simulink model "BaseEngineController_LS"  (Simulink 7.7)
settings: Solver=FixedStepDiscrete  StartTime=0.0  StopTime=10.0  RelTol=1e-3
PreLoadFcn:
  | try, eval([bdroot '_setup']); catch, eval('model_setup', ''); end
InitFcn:
  | try, eval([bdroot '_setup']); catch, eval('model_setup', ''); end
undefined symbols (not defined in the file): ECU555, High, motohawk_build_version, motohawk_trunc_name, motohawk_vardec_config_group, motohawk_vardec_path, True
libraries: MotoHawk_lib x1418, motohawk_control_primitives_lib x183, motohawk_engine_lib x32, simulink x21, motohawk_annotations_lib x9, AutoDoc_lib x8, simulink_extras x4, motohawk_ccp_examples_lib x1, motohawk_control_primitives_motoshare_lib x1
(part 6 of 27)

== system BaseEngineController_LS/Foreground/Control/Diagnostics/MAP Fault Logic ==
  Sensors : Inport
  Add : Sum  Inputs=+-
  Bus Selector : BusSelector  OutputSignals=RawProcessed.EngineState
  Bus Selector1 : BusSelector  OutputSignals=RawProcessed.TPS
  Bus Selector2 : BusSelector  OutputSignals=RawProcessed.TPS
  Bus Selector3 : BusSelector  OutputSignals=RawProcessed.TPS
  Bus Selector4 : BusSelector  OutputSignals=Raw.LinearSensors.MAP_Angular
  Bus Selector5 : BusSelector  OutputSignals=Raw.LinearSensors.MAP_Angular
  Bus Selector6 : BusSelector  OutputSignals=AirCalcs.Baro,Raw.LinearSensors.MAP_Angular
  Logical Operator1 : Logic  Operator=OR  Inputs=6  AllPortsSameDT=off  OutDataTypeStr=boolean
  Logical Operator2 : Logic  Inputs=4  AllPortsSameDT=off  OutDataTypeStr=boolean
  Logical Operator3 : Logic  Operator=NOT  Inputs=3  AllPortsSameDT=off  OutDataTypeStr=boolean
  Logical Operator4 : Logic  Inputs=4  AllPortsSameDT=off  OutDataTypeStr=boolean
  Logical Operator5 : Logic  Inputs=4  AllPortsSameDT=off  OutDataTypeStr=boolean
  Relational Operator1 : RelationalOperator  Operator=>  OutDataTypeStr=boolean
  Relational Operator{2..3,7..8} (4 alike) : RelationalOperator  Operator=<  OutDataTypeStr=boolean
  Relational Operator4 : RelationalOperator  Operator=>  OutDataTypeStr=boolean
  Run State : motohawk_control_primitives_lib/CompareTo  SystemSampleTime=-1  op===  val=3
  motohawk_calibration2 : MotoHawk_lib/Calibration & Probing Blocks/motohawk_calibration  nam='MAP_IR_TPS_CL'  val=50  storage=Calibration  show_more=on  name_source=Use Parameter  data_type=double  read_level=1  write_level=1  ovr_cals=on  view_as=Number  enum_struct={'Disabled', 'Enabled'}  vector_style=Wide Row  use_help_units=on  help="'In-range MAP fault logic.  Maximum throttle position, below which MAP should be less than MAP_IR_HI'"  units='%'  use_header_enum=off  row_header_enum={}  col_header_enum={}  use_min_max=off  min_val=0  max_val=inf  use_precision=off  precision=''  gain=1  offset=0  exp=1  use_mototune_group=on  mototune_group=motohawk_vardec_path(gcb)
  motohawk_calibration4 : MotoHawk_lib/Calibration & Probing Blocks/motohawk_calibration  nam='MAP_IR_HI'  val=50  storage=Calibration  show_more=on  name_source=Use Parameter  data_type=double  read_level=1  write_level=1  ovr_cals=on  view_as=Number  enum_struct={'Disabled', 'Enabled'}  vector_style=Wide Row  use_help_units=on  help='In-range MAP fault logic. Maximum value that MAP should not exceed with closed throttle and engine running'  units='kPa'  use_header_enum=off  row_header_enum={}  col_header_enum={}  use_min_max=off  min_val=0  max_val=inf  use_precision=off  precision=''  gain=1  offset=0  exp=1  use_mototune_group=on  mototune_group=motohawk_vardec_path(gcb)
  motohawk_calibration5 : MotoHawk_lib/Calibration & Probing Blocks/motohawk_calibration  nam='MAP_IR_LO'  val=50  storage=Calibration  show_more=on  name_source=Use Parameter  data_type=double  read_level=1  write_level=1  ovr_cals=on  view_as=Number  enum_struct={'Disabled', 'Enabled'}  vector_style=Wide Row  use_help_units=on  help='In-range MAP fault logic. Minimum value that MAP should not be less than with open throttle and engine running'  units='kPa'  use_header_enum=off  row_header_enum={}  col_header_enum={}  use_min_max=off  min_val=0  max_val=inf  use_precision=off  precision=''  gain=1  offset=0  exp=1  use_mototune_group=on  mototune_group=motohawk_vardec_path(gcb)
  motohawk_calibration6 : MotoHawk_lib/Calibration & Probing Blocks/motohawk_calibration  nam='MAP_IR_TPS_OP'  val=50  storage=Calibration  show_more=on  name_source=Use Parameter  data_type=double  read_level=1  write_level=1  ovr_cals=on  view_as=Number  enum_struct={'Disabled', 'Enabled'}  vector_style=Wide Row  use_help_units=on  help="'In-range MAP fault logic.  Minimum throttle position, above which MAP should be greater than MAP_IR_LO'"  units='%'  use_header_enum=off  row_header_enum={}  col_header_enum={}  use_min_max=off  min_val=0  max_val=inf  use_precision=off  precision=''  gain=1  offset=0  exp=1  use_mototune_group=on  mototune_group=motohawk_vardec_path(gcb)
  motohawk_calibration7 : MotoHawk_lib/Calibration & Probing Blocks/motohawk_calibration  nam='MAP_STUCK'  val=50  storage=Calibration  show_more=on  name_source=Use Parameter  data_type=double  read_level=1  write_level=1  ovr_cals=on  view_as=Number  enum_struct={'Disabled', 'Enabled'}  vector_style=Wide Row  use_help_units=on  help="'In-range MAP fault logic.  Minimum difference between MAP and BARO with throttle closed. If less than this, a fault exists'"  units='kPa'  use_header_enum=off  row_header_enum={}  col_header_enum={}  use_min_max=off  min_val=0  max_val=inf  use_precision=off  precision=''  gain=1  offset=0  exp=1  use_mototune_group=on  mototune_group=motohawk_vardec_path(gcb)
  motohawk_calibration8 : MotoHawk_lib/Calibration & Probing Blocks/motohawk_calibration  nam='MAP_TPS_STUCK'  val=50  storage=Calibration  show_more=on  name_source=Use Parameter  data_type=double  read_level=1  write_level=1  ovr_cals=on  view_as=Number  enum_struct={'Disabled', 'Enabled'}  vector_style=Wide Row  use_help_units=on  help="'In-range MAP fault logic.  Maximum throttle position, below\twhich MAP should be less than BARO'"  units='%'  use_header_enum=off  row_header_enum={}  col_header_enum={}  use_min_max=off  min_val=0  max_val=inf  use_precision=off  precision=''  gain=1  offset=0  exp=1  use_mototune_group=on  mototune_group=motohawk_vardec_path(gcb)
  motohawk_fault_def1 : MotoHawk_lib/Fault Management Blocks/motohawk_fault_def  nam='MAP_IR_HI'  mode=Enabled  id=[]  x=25  y=50  input_suspected=on  indeterminate=off  increment_xy=on  downsample_count=1  ovr_cals=on  ovr_actions=on  show_actions=off  action1_name=''  action1_cond=(None)  action2_name=''  action2_cond=(None)  action3_name=''  action3_cond=(None)  action4_name=''  action4_cond=(None)
  motohawk_fault_def2 : MotoHawk_lib/Fault Management Blocks/motohawk_fault_def  nam='MAP_IR_LO'  mode=Enabled  id=[]  x=25  y=50  input_suspected=on  indeterminate=off  increment_xy=on  downsample_count=1  ovr_cals=on  ovr_actions=on  show_actions=off  action1_name=''  action1_cond=(None)  action2_name=''  action2_cond=(None)  action3_name=''  action3_cond=(None)  action4_name=''  action4_cond=(None)
  motohawk_fault_def3 : MotoHawk_lib/Fault Management Blocks/motohawk_fault_def  nam='MAP_STICKING'  mode=Enabled  id=[]  x=25  y=50  input_suspected=on  indeterminate=off  increment_xy=on  downsample_count=1  ovr_cals=on  ovr_actions=on  show_actions=off  action1_name=''  action1_cond=(None)  action2_name=''  action2_cond=(None)  action3_name=''  action3_cond=(None)  action4_name=''  action4_cond=(None)
  motohawk_fault_status : MotoHawk_lib/Fault Management Blocks/motohawk_fault_status  source=Lookup By Name  nam='TPS1RangeHigh'  status=Active
  motohawk_fault_status1 : MotoHawk_lib/Fault Management Blocks/motohawk_fault_status  source=Lookup By Name  nam='TPS2RangeHigh'  status=Active
  motohawk_fault_status2 : MotoHawk_lib/Fault Management Blocks/motohawk_fault_status  source=Lookup By Name  nam='TPS1RangeLow'  status=Active
  motohawk_fault_status3 : MotoHawk_lib/Fault Management Blocks/motohawk_fault_status  source=Lookup By Name  nam='TPS2RangeLow'  status=Active
  motohawk_fault_status4 : MotoHawk_lib/Fault Management Blocks/motohawk_fault_status  source=Lookup By Name  nam='MAPRangeLow'  status=Active
  motohawk_fault_status5 : MotoHawk_lib/Fault Management Blocks/motohawk_fault_status  source=Lookup By Name  nam='MAPRangeHigh'  status=Active
  wires:
  Logical Operator5/1 -> motohawk_fault_def3/1
  Logical Operator2/1 -> motohawk_fault_def2/1
  Logical Operator4/1 -> motohawk_fault_def1/1
  Bus Selector6/2 -> Add/2  "<MAP_Angular>"
  Bus Selector6/1 -> Add/1  "<Baro>"
  Add/1 -> Relational Operator8/1
  motohawk_calibration7/1 -> Relational Operator8/2
  Relational Operator8/1 -> Logical Operator5/4
  Bus Selector1/1 -> Relational Operator7/1  "<TPS>"
  Relational Operator7/1 -> Logical Operator5/3
  motohawk_calibration8/1 -> Relational Operator7/2
  Bus Selector5/1 -> Relational Operator2/1  "<MAP_Angular>"
  motohawk_calibration5/1 -> Relational Operator2/2
  Relational Operator2/1 -> Logical Operator2/4
  Bus Selector2/1 -> Relational Operator1/1  "<TPS>"
  Relational Operator1/1 -> Logical Operator2/3
  motohawk_calibration6/1 -> Relational Operator1/2
  Sensors/1 -> Bus Selector6/1, Bus Selector1/1, Bus Selector5/1, Bus Selector2/1, Bus Selector4/1, Bus Selector3/1, Bus Selector/1
  Bus Selector4/1 -> Relational Operator4/1  "<MAP_Angular>"
  motohawk_calibration4/1 -> Relational Operator4/2
  Relational Operator4/1 -> Logical Operator4/4
  Bus Selector3/1 -> Relational Operator3/1  "<TPS>"
  Relational Operator3/1 -> Logical Operator4/3
  motohawk_calibration2/1 -> Relational Operator3/2
  Run State/1 -> Logical Operator5/2, Logical Operator2/2, Logical Operator4/2
  Logical Operator3/1 -> Logical Operator5/1, Logical Operator2/1, Logical Operator4/1
  Logical Operator1/1 -> Logical Operator3/1
  motohawk_fault_status4/1 -> Logical Operator1/6
  motohawk_fault_status5/1 -> Logical Operator1/5
  motohawk_fault_status3/1 -> Logical Operator1/4
  motohawk_fault_status2/1 -> Logical Operator1/3
  motohawk_fault_status1/1 -> Logical Operator1/2
  motohawk_fault_status/1 -> Logical Operator1/1
  Bus Selector/1 -> Run State/1  "<EngineState>"

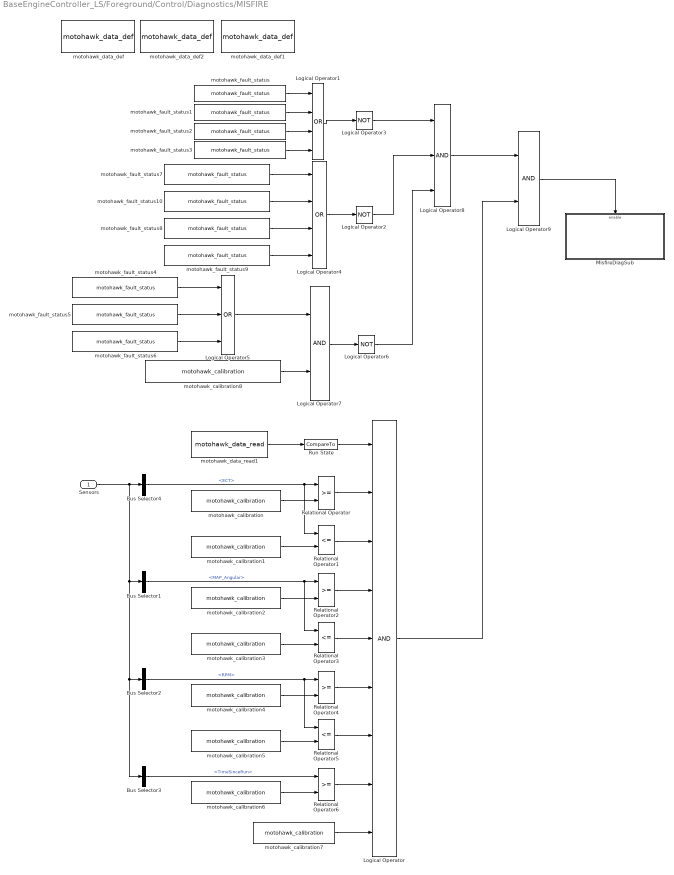
== system BaseEngineController_LS/Foreground/Control/Diagnostics/MISFIRE ==
  Sensors : Inport
  Bus Selector1 : BusSelector  OutputSignals=Raw.LinearSensors.MAP_Angular
  Bus Selector2 : BusSelector  OutputSignals=Raw.RPM
  Bus Selector3 : BusSelector  OutputSignals=RawProcessed.TimeSinceRun
  Bus Selector4 : BusSelector  OutputSignals=Raw.NonLinearSensors.ECT
  Logical Operator : Logic  Inputs=9  AllPortsSameDT=off  OutDataTypeStr=boolean
  Logical Operator1 : Logic  Operator=OR  Inputs=4  AllPortsSameDT=off  OutDataTypeStr=boolean
  Logical Operator2 : Logic  Operator=NOT  Inputs=3  AllPortsSameDT=off  OutDataTypeStr=boolean
  Logical Operator3 : Logic  Operator=NOT  Inputs=3  AllPortsSameDT=off  OutDataTypeStr=boolean
  Logical Operator4 : Logic  Operator=OR  Inputs=4  AllPortsSameDT=off  OutDataTypeStr=boolean
  Logical Operator5 : Logic  Operator=OR  Inputs=3  AllPortsSameDT=off  OutDataTypeStr=boolean
  Logical Operator6 : Logic  Operator=NOT  Inputs=3  AllPortsSameDT=off  OutDataTypeStr=boolean
  Logical Operator7 : Logic  AllPortsSameDT=off  OutDataTypeStr=boolean
  Logical Operator8 : Logic  Inputs=3  AllPortsSameDT=off  OutDataTypeStr=boolean
  Logical Operator9 : Logic  AllPortsSameDT=off  OutDataTypeStr=boolean
  MisfireDiagSub : Subsystem  TreatAsAtomicUnit=on
  Relational Operator{,2,4,6} (4 alike) : RelationalOperator  OutDataTypeStr=boolean
  Relational Operator1 : RelationalOperator  Operator=<=  OutDataTypeStr=boolean
  Relational Operator3 : RelationalOperator  Operator=<=  OutDataTypeStr=boolean
  Relational Operator5 : RelationalOperator  Operator=<=  OutDataTypeStr=boolean
  Run State : motohawk_control_primitives_lib/CompareTo  SystemSampleTime=-1  op===  val=3
  motohawk_calibration : MotoHawk_lib/Calibration & Probing Blocks/motohawk_calibration  nam='MisfireDiag_ECTLowEnbl'  val=-40  storage=Calibration  show_more=on  name_source=Use Parameter  data_type=int16  read_level=1  write_level=1  ovr_cals=on  view_as=Number  enum_struct={'Disabled', 'Enabled'}  vector_style=Wide Row  use_help_units=off  help=''  units=''  use_header_enum=off  row_header_enum={}  col_header_enum={}  use_min_max=off  min_val=-inf  max_val=inf  use_precision=off  precision=''  gain=1  offset=0  exp=1  use_mototune_group=off  mototune_group=motohawk_vardec_path(gcb)
  motohawk_calibration1 : MotoHawk_lib/Calibration & Probing Blocks/motohawk_calibration  nam='MisfireDiag_ECTHighEnbl'  val=150  storage=Calibration  show_more=on  name_source=Use Parameter  data_type=int16  read_level=1  write_level=1  ovr_cals=on  view_as=Number  enum_struct={'Disabled', 'Enabled'}  vector_style=Wide Row  use_help_units=off  help=''  units=''  use_header_enum=off  row_header_enum={}  col_header_enum={}  use_min_max=off  min_val=-inf  max_val=inf  use_precision=off  precision=''  gain=1  offset=0  exp=1  use_mototune_group=off  mototune_group=motohawk_vardec_path(gcb)
  motohawk_calibration2 : MotoHawk_lib/Calibration & Probing Blocks/motohawk_calibration  nam='MisfireDiag_MAPLowEnbl'  val=0  storage=Calibration  show_more=on  name_source=Use Parameter  data_type=int16  read_level=1  write_level=1  ovr_cals=on  view_as=Number  enum_struct={'Disabled', 'Enabled'}  vector_style=Wide Row  use_help_units=off  help=''  units=''  use_header_enum=off  row_header_enum={}  col_header_enum={}  use_min_max=off  min_val=-inf  max_val=inf  use_precision=off  precision=''  gain=1  offset=0  exp=1  use_mototune_group=off  mototune_group=motohawk_vardec_path(gcb)
  motohawk_calibration3 : MotoHawk_lib/Calibration & Probing Blocks/motohawk_calibration  nam='MisfireDiag_MAPHighEnbl'  val=150  storage=Calibration  show_more=on  name_source=Use Parameter  data_type=int16  read_level=1  write_level=1  ovr_cals=on  view_as=Number  enum_struct={'Disabled', 'Enabled'}  vector_style=Wide Row  use_help_units=off  help=''  units=''  use_header_enum=off  row_header_enum={}  col_header_enum={}  use_min_max=off  min_val=-inf  max_val=inf  use_precision=off  precision=''  gain=1  offset=0  exp=1  use_mototune_group=off  mototune_group=motohawk_vardec_path(gcb)
  motohawk_calibration4 : MotoHawk_lib/Calibration & Probing Blocks/motohawk_calibration  nam='MisfireDiag_RPMLowEnbl'  val=0  storage=Calibration  show_more=on  name_source=Use Parameter  data_type=int16  read_level=1  write_level=1  ovr_cals=on  view_as=Number  enum_struct={'Disabled', 'Enabled'}  vector_style=Wide Row  use_help_units=off  help=''  units=''  use_header_enum=off  row_header_enum={}  col_header_enum={}  use_min_max=off  min_val=-inf  max_val=inf  use_precision=off  precision=''  gain=1  offset=0  exp=1  use_mototune_group=off  mototune_group=motohawk_vardec_path(gcb)
  motohawk_calibration5 : MotoHawk_lib/Calibration & Probing Blocks/motohawk_calibration  nam='MisfireDiag_RPMHighEnbl'  val=10000  storage=Calibration  show_more=on  name_source=Use Parameter  data_type=int16  read_level=1  write_level=1  ovr_cals=on  view_as=Number  enum_struct={'Disabled', 'Enabled'}  vector_style=Wide Row  use_help_units=off  help=''  units=''  use_header_enum=off  row_header_enum={}  col_header_enum={}  use_min_max=off  min_val=-inf  max_val=inf  use_precision=off  precision=''  gain=1  offset=0  exp=1  use_mototune_group=off  mototune_group=motohawk_vardec_path(gcb)
  motohawk_calibration6 : MotoHawk_lib/Calibration & Probing Blocks/motohawk_calibration  nam='MisfireDiag_TimeSinceRunEnbl'  val=3  storage=Calibration  show_more=on  name_source=Use Parameter  data_type=int16  read_level=1  write_level=1  ovr_cals=on  view_as=Number  enum_struct={'Disabled', 'Enabled'}  vector_style=Wide Row  use_help_units=off  help=''  units=''  use_header_enum=off  row_header_enum={}  col_header_enum={}  use_min_max=off  min_val=-inf  max_val=inf  use_precision=off  precision=''  gain=1  offset=0  exp=1  use_mototune_group=off  mototune_group=motohawk_vardec_path(gcb)
  motohawk_calibration7 : MotoHawk_lib/Calibration & Probing Blocks/motohawk_calibration  nam='MisfireDiag_Enbl'  val=0  storage=Calibration  show_more=on  name_source=Use Parameter  data_type=boolean  read_level=1  write_level=1  ovr_cals=on  view_as=Enumeration  enum_struct={'Disabled', 'Enabled'}  vector_style=Wide Row  use_help_units=off  help=''  units=''  use_header_enum=off  row_header_enum={}  col_header_enum={}  use_min_max=off  min_val=-inf  max_val=inf  use_precision=off  precision=''  gain=1  offset=0  exp=1  use_mototune_group=off  mototune_group=motohawk_vardec_path(gcb)
  motohawk_calibration8 : MotoHawk_lib/Calibration & Probing Blocks/motohawk_calibration  nam='MisfireDiag_MAPIRDiagEnable'  val=0  storage=Calibration  show_more=on  name_source=Use Parameter  data_type=boolean  read_level=1  write_level=1  ovr_cals=on  view_as=Enumeration  enum_struct={'Disabled', 'Enabled'}  vector_style=Wide Row  use_help_units=off  help=''  units=''  use_header_enum=off  row_header_enum={}  col_header_enum={}  use_min_max=off  min_val=-inf  max_val=inf  use_precision=off  precision=''  gain=1  offset=0  exp=1  use_mototune_group=off  mototune_group=motohawk_vardec_path(gcb)
  motohawk_data_def : MotoHawk_lib/Data Storage Blocks/motohawk_data_def  nam='MisfireDiag_StartRPM'  container_nam=''  data=[0,0,0,0,0,0,0,0]  typ=uint16  struct_nam='MyStruct'  storage=Volatile  outputRef=off  use_vardec=off  window=Display  read_level=1  write_level=1  ovr_cals=on  view_as=Number  enum_struct={'Disabled', 'Enabled'}  vector_style=Wide Row  use_help_units=off  help=''  units=''  use_header_enum=off  row_header_enum=''  col_header_enum=''  use_min_max=off  min_val=-inf  max_val=inf  use_precision=off  precision=''  gain=1  offset=0  exp=1  use_mototune_group=off  mototune_group=motohawk_vardec_path(gcb)  eval_name=MyData  data_stores=motohawk_sfun_data_def_data_stores  struct_instances=motohawk_sfun_data_def_struct_instances  vardecs=motohawk_sfun_data_def_vardecs
  motohawk_data_def1 : MotoHawk_lib/Data Storage Blocks/motohawk_data_def  nam='MisfireDiag_RPMDR'  container_nam=''  data=[0,0,0,0,0,0,0,0]  typ=boolean  struct_nam='MyStruct'  storage=Volatile  outputRef=off  use_vardec=off  window=Display  read_level=1  write_level=1  ovr_cals=on  view_as=Number  enum_struct={'Disabled', 'Enabled'}  vector_style=Wide Row  use_help_units=off  help=''  units=''  use_header_enum=off  row_header_enum=''  col_header_enum=''  use_min_max=off  min_val=-inf  max_val=inf  use_precision=off  precision=''  gain=1  offset=0  exp=1  use_mototune_group=off  mototune_group=motohawk_vardec_path(gcb)  eval_name=MyData  data_stores=motohawk_sfun_data_def_data_stores  struct_instances=motohawk_sfun_data_def_struct_instances  vardecs=motohawk_sfun_data_def_vardecs
  motohawk_data_def2 : MotoHawk_lib/Data Storage Blocks/motohawk_data_def  nam='MisfireDiag_StopRPM'  container_nam=''  data=[0,0,0,0,0,0,0,0]  typ=uint16  struct_nam='MyStruct'  storage=Volatile  outputRef=off  use_vardec=off  window=Display  read_level=1  write_level=1  ovr_cals=on  view_as=Number  enum_struct={'Disabled', 'Enabled'}  vector_style=Wide Row  use_help_units=off  help=''  units=''  use_header_enum=off  row_header_enum=''  col_header_enum=''  use_min_max=off  min_val=-inf  max_val=inf  use_precision=off  precision=''  gain=1  offset=0  exp=1  use_mototune_group=off  mototune_group=motohawk_vardec_path(gcb)  eval_name=MyData  data_stores=motohawk_sfun_data_def_data_stores  struct_instances=motohawk_sfun_data_def_struct_instances  vardecs=motohawk_sfun_data_def_vardecs
  motohawk_data_read1 : MotoHawk_lib/Data Storage Blocks/motohawk_data_read  source=Lookup By Name  structure=Scalar  operation=Read entire data structure at once  sz_vec=4  sz_row=2  sz_col=3  typ=uint8  nam='EngineState'  checkNull=on  struct_inst_name='Struct1'  struct_nam='MyStruct'
  motohawk_fault_status : MotoHawk_lib/Fault Management Blocks/motohawk_fault_status  source=Lookup By Name  nam='ECTRangeHigh'  status=Active
  motohawk_fault_status1 : MotoHawk_lib/Fault Management Blocks/motohawk_fault_status  source=Lookup By Name  nam='ECTRangeLow'  status=Active
  motohawk_fault_status10 : MotoHawk_lib/Fault Management Blocks/motohawk_fault_status  source=Lookup By Name  nam='CrankEdgesFault'  status=Active
  motohawk_fault_status2 : MotoHawk_lib/Fault Management Blocks/motohawk_fault_status  source=Lookup By Name  nam='MAPRangeHigh'  status=Active
  motohawk_fault_status3 : MotoHawk_lib/Fault Management Blocks/motohawk_fault_status  source=Lookup By Name  nam='MAPRangeLow'  status=Active
  motohawk_fault_status4 : MotoHawk_lib/Fault Management Blocks/motohawk_fault_status  source=Lookup By Name  nam='MAP_IR_HI'  status=Active
  motohawk_fault_status5 : MotoHawk_lib/Fault Management Blocks/motohawk_fault_status  source=Lookup By Name  nam='MAP_IR_LO'  status=Active
  motohawk_fault_status6 : MotoHawk_lib/Fault Management Blocks/motohawk_fault_status  source=Lookup By Name  nam='MAP_STICKING'  status=Active
  motohawk_fault_status7 : MotoHawk_lib/Fault Management Blocks/motohawk_fault_status  source=Lookup By Name  nam='CrankSyncFault'  status=Active
  motohawk_fault_status8 : MotoHawk_lib/Fault Management Blocks/motohawk_fault_status  source=Lookup By Name  nam='CamEdgesFault'  status=Active
  motohawk_fault_status9 : MotoHawk_lib/Fault Management Blocks/motohawk_fault_status  source=Lookup By Name  nam='CamSyncFault'  status=Active
  wires:
  Sensors/1 -> Bus Selector4/1, Bus Selector1/1, Bus Selector2/1, Bus Selector3/1
  motohawk_data_read1/1 -> Run State/1
  Bus Selector4/1 -> Relational Operator/1, Relational Operator1/1  "<ECT>"
  motohawk_calibration/1 -> Relational Operator/2
  motohawk_calibration1/1 -> Relational Operator1/2
  Bus Selector1/1 -> Relational Operator2/1, Relational Operator3/1  "<MAP_Angular>"
  motohawk_calibration2/1 -> Relational Operator2/2
  motohawk_calibration3/1 -> Relational Operator3/2
  Bus Selector2/1 -> Relational Operator4/1, Relational Operator5/1  "<RPM>"
  motohawk_calibration4/1 -> Relational Operator4/2
  motohawk_calibration5/1 -> Relational Operator5/2
  Bus Selector3/1 -> Relational Operator6/1  "<TimeSinceRun>"
  motohawk_calibration6/1 -> Relational Operator6/2
  Relational Operator6/1 -> Logical Operator/8
  Relational Operator5/1 -> Logical Operator/7
  Run State/1 -> Logical Operator/1
  Relational Operator/1 -> Logical Operator/2
  Relational Operator1/1 -> Logical Operator/3
  Relational Operator2/1 -> Logical Operator/4
  Relational Operator3/1 -> Logical Operator/5
  Relational Operator4/1 -> Logical Operator/6
  motohawk_calibration7/1 -> Logical Operator/9
  motohawk_fault_status/1 -> Logical Operator1/1
  motohawk_fault_status1/1 -> Logical Operator1/2
  Logical Operator1/1 -> Logical Operator3/1
  motohawk_fault_status4/1 -> Logical Operator5/1
  motohawk_fault_status5/1 -> Logical Operator5/2
  motohawk_fault_status6/1 -> Logical Operator5/3
  Logical Operator5/1 -> Logical Operator7/1
  Logical Operator7/1 -> Logical Operator6/1
  motohawk_calibration8/1 -> Logical Operator7/2
  motohawk_fault_status7/1 -> Logical Operator4/1
  Logical Operator4/1 -> Logical Operator2/1
  motohawk_fault_status10/1 -> Logical Operator4/2
  motohawk_fault_status8/1 -> Logical Operator4/3
  motohawk_fault_status9/1 -> Logical Operator4/4
  motohawk_fault_status2/1 -> Logical Operator1/3
  motohawk_fault_status3/1 -> Logical Operator1/4
  Logical Operator3/1 -> Logical Operator8/1
  Logical Operator2/1 -> Logical Operator8/2
  Logical Operator6/1 -> Logical Operator8/3
  Logical Operator8/1 -> Logical Operator9/1
  Logical Operator/1 -> Logical Operator9/2
  Logical Operator9/1 -> MisfireDiagSub/Enable

== system BaseEngineController_LS/Foreground/Control/Diagnostics/O2 Smart Sensor ==
  Sensors : Inport
  DesEquivRatio : Inport  Port=2
  Bank2Bank : Subsystem
  SensorStatus : Subsystem
  SensorVolt : Subsystem
  wires:
  Sensors/1 -> SensorVolt/1(Sensors), SensorStatus/1(Sensors), Bank2Bank/1(Sensors)
  DesEquivRatio/1 -> Bank2Bank/2(DesEquivRatio)

== system BaseEngineController_LS/Foreground/Control/Diagnostics/Overspeed Protection ==
  RPM : Inport
  BaseRevLimit : Subsystem
  Data Type Conversion : DataTypeConversion  OutDataTypeStr=int16
  Logical Operator1 : Logic  AllPortsSameDT=off  OutDataTypeStr=boolean
  Logical Operator2 : Logic  AllPortsSameDT=off  OutDataTypeStr=boolean
  Logical Operator3 : Logic  AllPortsSameDT=off  OutDataTypeStr=boolean
  Logical Operator4 : Logic  Operator=OR  Inputs=4  AllPortsSameDT=off  OutDataTypeStr=boolean
  Logical Operator5 : Logic  Operator=NOT  Inputs=3  AllPortsSameDT=off  OutDataTypeStr=boolean
  motohawk_fault_def1 : MotoHawk_lib/Fault Management Blocks/motohawk_fault_def  nam='SoftOverspeed'  mode=Enabled  id=[]  x=5  y=10  input_suspected=on  indeterminate=off  increment_xy=on  downsample_count=1  ovr_cals=on  ovr_actions=on  show_actions=off  action1_name=''  action1_cond=(None)  action2_name=''  action2_cond=(None)  action3_name=''  action3_cond=(None)  action4_name=''  action4_cond=(None)
  motohawk_fault_def2 : MotoHawk_lib/Fault Management Blocks/motohawk_fault_def  nam='MediumOverspeed'  mode=Enabled  id=[]  x=5  y=10  input_suspected=on  indeterminate=off  increment_xy=on  downsample_count=1  ovr_cals=on  ovr_actions=on  show_actions=off  action1_name=''  action1_cond=(None)  action2_name=''  action2_cond=(None)  action3_name=''  action3_cond=(None)  action4_name=''  action4_cond=(None)
  motohawk_fault_def3 : MotoHawk_lib/Fault Management Blocks/motohawk_fault_def  nam='HardOverspeed'  mode=Enabled  id=[]  x=5  y=10  input_suspected=on  indeterminate=off  increment_xy=on  downsample_count=1  ovr_cals=on  ovr_actions=on  show_actions=off  action1_name=''  action1_cond=(None)  action2_name=''  action2_cond=(None)  action3_name=''  action3_cond=(None)  action4_name=''  action4_cond=(None)
  motohawk_fault_status1 : MotoHawk_lib/Fault Management Blocks/motohawk_fault_status  source=Lookup By Name  nam='CrankSyncFault'  status=Active
  motohawk_fault_status2 : MotoHawk_lib/Fault Management Blocks/motohawk_fault_status  source=Lookup By Name  nam='CamEdgesFault'  status=Active
  motohawk_fault_status3 : MotoHawk_lib/Fault Management Blocks/motohawk_fault_status  source=Lookup By Name  nam='CamSyncFault'  status=Active
  motohawk_fault_status4 : MotoHawk_lib/Fault Management Blocks/motohawk_fault_status  source=Lookup By Name  nam='CrankEdgesFault'  status=Active
  wires:
  RPM/1 -> Data Type Conversion/1
  Data Type Conversion/1 -> BaseRevLimit/1(RPM)
  BaseRevLimit/1(Soft) -> Logical Operator1/2
  BaseRevLimit/2(Medium) -> Logical Operator2/2
  BaseRevLimit/3(Hard) -> Logical Operator3/2
  Logical Operator1/1 -> motohawk_fault_def1/1
  Logical Operator2/1 -> motohawk_fault_def2/1
  Logical Operator3/1 -> motohawk_fault_def3/1
  motohawk_fault_status1/1 -> Logical Operator4/1
  Logical Operator4/1 -> Logical Operator5/1
  motohawk_fault_status4/1 -> Logical Operator4/2
  motohawk_fault_status2/1 -> Logical Operator4/3
  motohawk_fault_status3/1 -> Logical Operator4/4
  Logical Operator5/1 -> Logical Operator1/1, Logical Operator2/1, Logical Operator3/1

== system BaseEngineController_LS/Foreground/Control/Diagnostics/Wrong Fuel Pressure Fault Logic ==
  Sensors : Inport
  Bus Selector1 : BusSelector  OutputSignals=Raw.Digital.ESTOP
  Bus Selector4 : BusSelector  OutputSignals=RawProcessed.FuelDeltaPressure
  Logical Operator1 : Logic  Operator=OR  Inputs=3  AllPortsSameDT=off  OutDataTypeStr=boolean
  Logical Operator2 : Logic  AllPortsSameDT=off  OutDataTypeStr=boolean
  Logical Operator3 : Logic  Operator=NOT  Inputs=3  AllPortsSameDT=off  OutDataTypeStr=boolean
  Logical Operator4 : Logic  AllPortsSameDT=off  OutDataTypeStr=boolean
  Relational Operator1 : RelationalOperator  Operator=<  OutDataTypeStr=boolean
  Relational Operator3 : RelationalOperator  Operator=>  OutDataTypeStr=boolean
  Sum3 : Sum  Inputs=+-  SaturateOnIntegerOverflow=on
  invert : Gain  Gain=-1  SaturateOnIntegerOverflow=on  OutDataTypeStr=Inherit: Same as input  ParamDataTypeStr=Inherit: Same as input
  motohawk_calibration2 : MotoHawk_lib/Calibration & Probing Blocks/motohawk_calibration  nam='FuelPres_DeltaTarget'  val=343  storage=Calibration  show_more=on  name_source=Use Parameter  data_type=double  read_level=1  write_level=1  ovr_cals=on  view_as=Number  enum_struct={'Disabled', 'Enabled'}  vector_style=Wide Row  use_help_units=on  help='Target fuel pressure delta across injector (rail - manifold)'  units='kPa'  use_header_enum=off  row_header_enum={}  col_header_enum={}  use_min_max=off  min_val=-inf  max_val=inf  use_precision=off  precision=''  gain=1  offset=0  exp=1  use_mototune_group=on  mototune_group=motohawk_vardec_path(gcb)
  motohawk_calibration3 : MotoHawk_lib/Calibration & Probing Blocks/motohawk_calibration  nam='FuelPres_DeltaTolerance'  val=25  storage=Calibration  show_more=on  name_source=Use Parameter  data_type=double  read_level=1  write_level=1  ovr_cals=on  view_as=Number  enum_struct={'Disabled', 'Enabled'}  vector_style=Wide Row  use_help_units=on  help='Target fuel pressure delta across injector (rail - manifold)'  units='kPa'  use_header_enum=off  row_header_enum={}  col_header_enum={}  use_min_max=off  min_val=-inf  max_val=inf  use_precision=off  precision=''  gain=1  offset=0  exp=1  use_mototune_group=on  mototune_group=motohawk_vardec_path(gcb)
  motohawk_fault_def1 : MotoHawk_lib/Fault Management Blocks/motohawk_fault_def  nam='FuelPresLow_Fault'  mode=Enabled  id=[]  x=25  y=50  input_suspected=on  indeterminate=off  increment_xy=on  downsample_count=1  ovr_cals=on  ovr_actions=on  show_actions=on  action1_name=''  action1_cond=(None)  action2_name=''  action2_cond=(None)  action3_name=''  action3_cond=(None)  action4_name=''  action4_cond=(None)
  motohawk_fault_def2 : MotoHawk_lib/Fault Management Blocks/motohawk_fault_def  nam='FuelPresHigh_Fault'  mode=Enabled  id=[]  x=25  y=50  input_suspected=on  indeterminate=off  increment_xy=on  downsample_count=1  ovr_cals=on  ovr_actions=on  show_actions=on  action1_name=''  action1_cond=(None)  action2_name=''  action2_cond=(None)  action3_name=''  action3_cond=(None)  action4_name=''  action4_cond=(None)
  motohawk_fault_status : MotoHawk_lib/Fault Management Blocks/motohawk_fault_status  source=Lookup By Name  nam='FuelPresRangeHigh'  status=Active
  motohawk_fault_status1 : MotoHawk_lib/Fault Management Blocks/motohawk_fault_status  source=Lookup By Name  nam='FuelPresRangeLow'  status=Active
  wires:
  Logical Operator4/1 -> motohawk_fault_def1/1
  Sensors/1 -> Bus Selector4/1, Bus Selector1/1
  Logical Operator3/1 -> Logical Operator4/1, Logical Operator2/1
  Logical Operator1/1 -> Logical Operator3/1
  motohawk_fault_status1/1 -> Logical Operator1/2
  motohawk_fault_status/1 -> Logical Operator1/1
  Relational Operator1/1 -> Logical Operator4/2
  Bus Selector4/1 -> Sum3/1  "<FuelDeltaPressure>"
  motohawk_calibration2/1 -> Sum3/2
  Sum3/1 -> Relational Operator1/1, Relational Operator3/1
  motohawk_calibration3/1 -> Relational Operator3/2, invert/1
  invert/1 -> Relational Operator1/2
  Logical Operator2/1 -> motohawk_fault_def2/1
  Relational Operator3/1 -> Logical Operator2/2
  Bus Selector1/1 -> Logical Operator1/3  "<ESTOP>"

== system BaseEngineController_LS/Foreground/Control/VirtualSensors/AirCalcs ==
  RawIndexes : Inport
  Raw : Inport  Port=2
  SSEngOpr : Inport  Port=3
  RawProcessed : Inport  Port=4
  Baro Stall State Delay : Stateflow chart  TreatAsAtomicUnit=on
  Bus Creator1 : BusCreator  Inputs=2
  Bus Selector1 : BusSelector  OutputSignals=LinearSensors.MAP_Angular,RPM,NonLinearSensors.IAT,Digital.MAF
  Bus Selector2 : BusSelector  OutputSignals=ECT09Idx
  Bus Selector3 : BusSelector  OutputSignals=IAT17Idx,RPM17Idx
  Bus Selector4 : BusSelector  OutputSignals=NonLinearSensors.ECT
  Bus Selector5 : BusSelector  OutputSignals=LinearSensors.MAP_Time_Raw
  Bus Selector6 : BusSelector  OutputSignals=TimeSinceRun,EngineState
  Capture Signal At Startup : Subsystem  AncestorBlock=motohawk_engine_lib/Capture Signal At Startup  TreatAsAtomicUnit=on  mask(Capture Signal At Startup){nam='Baro', count=5, units='kPa', grp=motohawk_vardec_path(gcb)}
      mask prompts: nam "Signal Name"; count "Number Of Samples To Average"; grp "MotoTune GroupString Name"
      mask init:
      | lbl = sprintf('CAPTURE IN STALL\nAverage of\nfirst %d samples', count);
      mask Display:
      | patch([0 0 1 1], [0 0.075 0.075 0], [230/255 0/255 0/255])
      | patch([0 0 1 1], [0.025 0.05 0.05 0.025], [150/255 0/255 0/255])
      | patch([0 0 1 1], [0 0.025 0.025 0], [0/255 0/255 0/255])
      | 
      | disp(lbl);
  Logical Operator : Logic  Operator=OR  AllPortsSameDT=off  OutDataTypeStr=boolean
  Running Baro Learn : Subsystem
  Saturation1 : Saturate  UpperLimit=inf  LowerLimit=1
  Speed Density - MAP Referenced - Adaptive : Subsystem  Description=|  AncestorBlock=motohawk_engine_lib/Speed Density - MAP Referenced - Adaptive
      | /* Name: PortPressRatio20IdxArr Unit:unitless ClassID:ORDARR StorageID:FLASH Access:RW4+RW3+NA2+NA1              
      |    TypeID:UINT2 Gain:0.0001 Min:0.0000 Max:6.5535 Format:5.4 UpdateID:REMOTE OrdLen:20 Group:"Engine Control | " 
      |    "Run | Airflow" Help:"Port pressure ratio index array. Used for speed-density flow computations." VardecSig:6E
      |    */                                                                                                            
      |                                                                                                                  
      | /* Name: RPM20IdxArr Unit:RPM20IdxArr ClassID:ORDARR StorageID:FLASH Access:RW4+RW3+NA2+NA1                      
      |    TypeID:UINT2 Gain:0.1 Min:0.0 Max:6553.0 Format:5.1 UpdateID:REMOTE OrdLen:20 Group:"Global "                 
      |    "Index Arrays | RPM" Help:"20 breakpoint RPM index array." VardecSig:5E */                                    
      |                                                                                                                  
      | /* Name: VolEffMap Unit:Unitless ClassID:MAP StorageID:FLASH Access:RW4+RW3+NA2+NA1 TypeID:UINT2                 
      |    Gain:0.0001 Min:0.00 Max:6.55 Format:6.2 UpdateID:REMOTE XOrdArr:PortPressRatio20IdxArr                       
      |    YOrdArr:RPM20IdxArr Group:"Engine Control | Run | Airflow" Help:"Engine volumetric efficency "                
      |    "map." VardecSig:61 */                                                                                        
      |                                                                                                                  
      | /* Name: IAT10IdxArr Unit:C ClassID:ORDARR StorageID:FLASH Access:RW4+RW3+NA2+NA1                                
      |    TypeID:SINT2 Gain:0.01 Min:-327.6800 Max:327.6700 Format:5.4 UpdateID:REMOTE OrdLen:10                        
      |    Group:"Engine Control | Run | Airflow" Help:"10 breakpoint intake air temperture index "                      
      |    "array." VardecSig:5C */                                                                                      
      |                                                                                                                  
      | /* Name: VETempCorrTbl ClassID:TBL StorageID:FLASH Access:RW4+RW3+NA2+NA1 TypeID:UINT2 Gain:0.0001 Min:0.00      
      |    Max:6.55 Format:4.2 UpdateID:REMOTE OrdArr:IAT10IdxArr Group:"Engine Control | Run | Airflow"                 
      |    Help:"Volumetric efficiency temperature correction table." VardecSig:6C */                                    
      |                                                                                                                  
      | /* Name: BaroPress10IdxArr Unit:C ClassID:ORDARR StorageID:FLASH Access:RW4+RW3+NA2+NA1                          
      |    TypeID:UINT2 Gain:0.01 Min:0.0000 Max:655.3500 Format:5.4 UpdateID:REMOTE OrdLen:10                           
      |    Group:"Engine Control | Run | Airflow" Help:"10 breakpoint barometric pressure index "                        
      |    "array." VardecSig:5C */                                                                                      
      |                                                                                                                  
      | /* Name: VEBaroCorrTbl ClassID:TBL StorageID:FLASH Access:RW4+RW3+NA2+NA1 TypeID:UINT2 Gain:0.0001 Min:0.00      
      |    Max:6.55 Format:4.2 UpdateID:REMOTE OrdArr:BaroPress10IdxArr Group:"Engine Control | Run | Airflow"           
      |    Help:"Volumetric efficiency barometric pressure correction table." VardecSig:6C */                            
      |                                                                                                                  
      | /* Name: CylSweptVol Unit:cm^3 ClassID:VAR StorageID:FLASH Access:RW4+RW3+NA2+NA1 TypeID:UINT2 Gain:0.1          
      |    Min:0.0 Max:6553.0 Format:5.1 UpdateID:REMOTE Group:"Engine Control | Run | Airflow" Help:"Cylinder swept "   
      |    "volume." VardecSig:6C */                                                                                     
      |                                                                                                                  
      | /* Name: MAFPort Unit:g/s ClassID:VAR StorageID:RAM Access:RO4+RO3+NA2+NA1 TypeID:UINT2 Gain:0.01                
      |    Min:0.00 Max:655.00 Format:5.2 UpdateID:BACKGND Group:"Engine Control | Run | Airflow" Help:"Total "          
      |    "ingested cylinder charge mass flow rate. The sum of all port flows. This values includes any EGR and "       
      |    "Purge mass flows." VardecSig:6A */                                                                           
      |                                                                                                                  
      | /* Name: CombEventsPerRev ClassID:VAR StorageID:FLASH Access:RW4+RW3+NA2+NA1 TypeID:UINT1 Gain:0.5 Min:0.5       
      |    Max:127.0 Format:4.1 UpdateID:REMOTE Group:"Engine Control | Run | Airflow" Help:"Number of conbustion "      
      |    "events per engine revolution. For example, for a four-stroke, eight cylinder engine the value would be 4."   
      |    VardecSig:6C */
      mask Description: Calculates air mass flow rate per cylinder. The estimated mass flow rate is that of the entire mixture: air, EGR and purge.
      mask Help: Given calibrations for the volumetric efficiency map, cylinder swept volume [cm3] and the VE temperature and pressure correction tables, the block calculates the air mass flow rate [g/s] per cylinder, given the barometric and manifold pressures [kPa], the manifold air temperature [C] and RPM.
      mask Display:
      | patch([0 0 1 1], 0.5*[0 0.075 0.075 0], [230/255 0/255 0/255])
      | patch([0 0 1 1], 0.5*[0.025 0.05 0.05 0.025], [150/255 0/255 0/255])
      | patch([0 0 1 1], 0.5*[0 0.025 0.025 0], [0/255 0/255 0/255])
      | 
      | disp('MAP-REFERENCED\nSPEED-DENSITY\nCOMPUTATION\n(adaptive)');
  motohawk_calibration : MotoHawk_lib/Calibration & Probing Blocks/motohawk_calibration  nam='BaroRunStallDelay'  val=4  storage=Calibration  show_more=on  name_source=Use Parameter  data_type=Inherit from 'Default Value'  read_level=1  write_level=1  ovr_cals=on  view_as=Number  enum_struct={'Disabled', 'Enabled'}  vector_style=Wide Row  use_help_units=on  help='Delay time after transitioning from Run to Stall before resampling baro.'  units='s'  use_header_enum=off  row_header_enum={}  col_header_enum={}  use_min_max=off  min_val=-inf  max_val=inf  use_precision=off  precision=''  gain=1  offset=0  exp=1  use_mototune_group=on  mototune_group=motohawk_vardec_path(gcb)
  motohawk_data_read1 : MotoHawk_lib/Data Storage Blocks/motohawk_data_read  source=Lookup By Name  structure=Scalar  operation=Read entire data structure at once  sz_vec=4  sz_row=2  sz_col=3  typ=uint8  nam='EngineState'  checkNull=on  struct_inst_name='Struct1'  struct_nam='MyStruct'
  motohawk_delta_time : MotoHawk_lib/Extra Development Blocks/motohawk_delta_time  samp_time=-1  init_val=.005  mode=Seconds (double)
  motohawk_override_rel : MotoHawk_lib/Calibration & Probing Blocks/motohawk_override_rel  SystemSampleTime=-1  parent_name='BARO'  show_more=on  name_source=Use Parameter  parent_read_level=1  parent_override_level=1  use_help_units=on  parent_help='Provides an override to the input by adding this amount to either the locked or running value'  parent_units='kPa'  use_min_max=off  parent_min=-inf  parent_max=inf  use_precision=off  parent_precision=''  parent_gain=1  parent_offset=0  parent_exp=1  use_mototune_group=on  parent_group=motohawk_vardec_path(gcb)
  motohawk_probe : MotoHawk_lib/Calibration & Probing Blocks/motohawk_probe  nam='BARO'  show_more=on  name_source=Use Parameter  read_level=1  view_as=Number  enum_struct={'Disabled', 'Enabled'}  vector_style=Wide Row  use_help_units=on  help=''  units='kPa'  use_header_enum=off  row_header_enum={}  col_header_enum={}  use_precision=off  precision=''  gain=1  offset=0  exp=1  use_mototune_group=on  mototune_group=motohawk_vardec_path(gcb)
  motohawk_probe1 : MotoHawk_lib/Calibration & Probing Blocks/motohawk_probe  nam='BaroDelayTime'  show_more=on  name_source=Use Parameter  read_level=1  view_as=Number  enum_struct={'Disabled', 'Enabled'}  vector_style=Wide Row  use_help_units=on  help=''  units='s'  use_header_enum=off  row_header_enum={}  col_header_enum={}  use_precision=off  precision=''  gain=1  offset=0  exp=1  use_mototune_group=on  mototune_group=motohawk_vardec_path(gcb)
  AirCalcs : Outport
  wires:
  Bus Selector5/1 -> Capture Signal At Startup/1(Signal_In), Running Baro Learn/2(MAP)  "<MAP_Time_Raw>"
  Bus Selector1/3 -> Speed Density - MAP Referenced - Adaptive/4(IAT [C])  "<IAT>"
  Raw/1 -> Bus Selector5/1, Bus Selector1/1, Bus Selector4/1
  RawIndexes/1 -> Bus Selector3/1, Bus Selector2/1
  Bus Selector3/1 -> Speed Density - MAP Referenced - Adaptive/6(IAT17Idx)  "<IAT17Idx>"
  Bus Selector3/2 -> Speed Density - MAP Referenced - Adaptive/7(RPMIdx)  "<RPM17Idx>"
  Bus Selector1/1 -> Speed Density - MAP Referenced - Adaptive/2(MAP [kPa])  "<MAP_Angular>"
  Bus Selector1/2 -> Speed Density - MAP Referenced - Adaptive/3(RPM)  "<RPM>"
  Bus Creator1/1 -> AirCalcs/1  "AirCalcs"
  Speed Density - MAP Referenced - Adaptive/1(MAF [g/s]) -> Bus Creator1/2  "MAFPort"
  motohawk_override_rel/1 -> motohawk_probe/1, Bus Creator1/1, Saturation1/1  "Baro"
  Capture Signal At Startup/1(Signal_KeyUp) -> motohawk_override_rel/1  "Baro"
  Saturation1/1 -> Speed Density - MAP Referenced - Adaptive/1(BARO [kPa])
  Bus Selector1/4 -> Speed Density - MAP Referenced - Adaptive/5(MAF_Sensor [g/s])  "<MAF>"
  motohawk_data_read1/1 -> Baro Stall State Delay/1(EngineState), Running Baro Learn/1(Eng State)
  motohawk_delta_time/1 -> Baro Stall State Delay/3(dT)
  motohawk_calibration/1 -> Baro Stall State Delay/2(TimeThresh)
  Baro Stall State Delay/1(Timer) -> motohawk_probe1/1
  SSEngOpr/1 -> Speed Density - MAP Referenced - Adaptive/8(SSEngOpr [bool])
  Bus Selector2/1 -> Speed Density - MAP Referenced - Adaptive/9(ECT09Idx)  "<ECT09Idx>"
  Bus Selector4/1 -> Speed Density - MAP Referenced - Adaptive/10(ECT [C])  "<ECT>"
  RawProcessed/1 -> Bus Selector6/1
  Bus Selector6/2 -> Speed Density - MAP Referenced - Adaptive/12(EngState)  "<EngineState>"
  Bus Selector6/1 -> Speed Density - MAP Referenced - Adaptive/11(TimeAfterRun [S])  "<TimeSinceRun>"
  Baro Stall State Delay/2(Enable) -> Logical Operator/1
  Logical Operator/1 -> Capture Signal At Startup/Enable
  Running Baro Learn/1(Enbl) -> Logical Operator/2
